simulink model "Monza"  (R2020a)
settings: Solver=FixedStepAuto  StartTime=0.0  StopTime=30  FixedStep=0.033  RelTol=1e-3
libraries: fuzblock x1, simulink x1
settings Model: Creator=jmpas  LastModifiedBy=jmpas

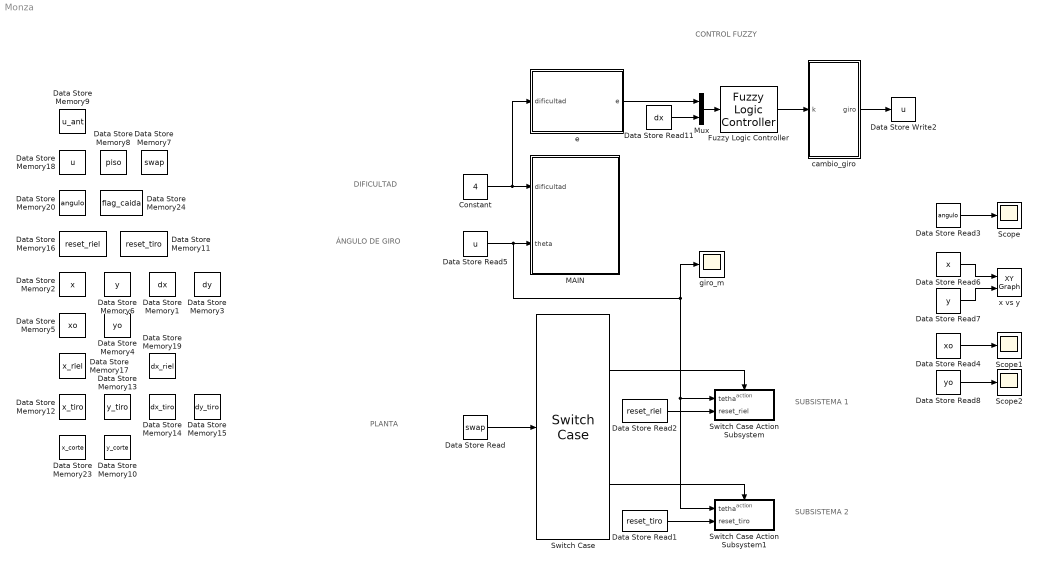
== system Monza ==
  note: CONTROL FUZZY
  note: DIFICULTAD
  note: ÁNGULO DE GIRO
  note: PLANTA
  note: SUBSISTEMA 1
  note: SUBSISTEMA 2
  " MAIN" : MATLAB Function  TreatAsAtomicUnit=on
  Constant : Constant  Value=4
  Data Store Memory1 : DataStoreMemory  DataStoreName=dx  ReadBeforeWriteMsg=warning  WriteAfterWriteMsg=warning  WriteAfterReadMsg=warning  ShowAdditionalParam=off  OutDataTypeStr=double
  Data Store Memory10 : DataStoreMemory  DataStoreName=y_corte  ReadBeforeWriteMsg=warning  WriteAfterWriteMsg=warning  WriteAfterReadMsg=warning  ShowAdditionalParam=off  OutDataTypeStr=double
  Data Store Memory11 : DataStoreMemory  DataStoreName=reset_tiro  ReadBeforeWriteMsg=warning  WriteAfterWriteMsg=warning  WriteAfterReadMsg=warning  ShowAdditionalParam=off  OutDataTypeStr=double
  Data Store Memory12 : DataStoreMemory  DataStoreName=x_tiro  ReadBeforeWriteMsg=warning  WriteAfterWriteMsg=warning  WriteAfterReadMsg=warning  ShowAdditionalParam=off  OutDataTypeStr=double
  Data Store Memory13 : DataStoreMemory  DataStoreName=y_tiro  ReadBeforeWriteMsg=warning  WriteAfterWriteMsg=warning  WriteAfterReadMsg=warning  ShowAdditionalParam=off  OutDataTypeStr=double
  Data Store Memory14 : DataStoreMemory  DataStoreName=dx_tiro  ReadBeforeWriteMsg=warning  WriteAfterWriteMsg=warning  WriteAfterReadMsg=warning  ShowAdditionalParam=off  OutDataTypeStr=double
  Data Store Memory15 : DataStoreMemory  DataStoreName=dy_tiro  ReadBeforeWriteMsg=warning  WriteAfterWriteMsg=warning  WriteAfterReadMsg=warning  ShowAdditionalParam=off  OutDataTypeStr=double
  Data Store Memory16 : DataStoreMemory  DataStoreName=reset_riel  ReadBeforeWriteMsg=warning  WriteAfterWriteMsg=warning  WriteAfterReadMsg=warning  ShowAdditionalParam=off  OutDataTypeStr=double
  Data Store Memory17 : DataStoreMemory  DataStoreName=x_riel  ReadBeforeWriteMsg=warning  WriteAfterWriteMsg=warning  WriteAfterReadMsg=warning  InitialValue=-0.11  ShowAdditionalParam=off  OutDataTypeStr=double
  Data Store Memory18 : DataStoreMemory  DataStoreName=u  ReadBeforeWriteMsg=warning  WriteAfterWriteMsg=warning  WriteAfterReadMsg=warning  InitialValue=-0.25  ShowAdditionalParam=off  OutDataTypeStr=double
  Data Store Memory19 : DataStoreMemory  DataStoreName=dx_riel  ReadBeforeWriteMsg=warning  WriteAfterWriteMsg=warning  WriteAfterReadMsg=warning  ShowAdditionalParam=off  OutDataTypeStr=double
  Data Store Memory2 : DataStoreMemory  DataStoreName=x  ReadBeforeWriteMsg=warning  WriteAfterWriteMsg=warning  WriteAfterReadMsg=warning  InitialValue=-0.11  ShowAdditionalParam=off  OutDataTypeStr=double
  Data Store Memory20 : DataStoreMemory  DataStoreName=angulo  ReadBeforeWriteMsg=warning  WriteAfterWriteMsg=warning  WriteAfterReadMsg=warning  InitialValue=-0.25  ShowAdditionalParam=off  OutDataTypeStr=double
  Data Store Memory23 : DataStoreMemory  DataStoreName=x_corte  ReadBeforeWriteMsg=warning  WriteAfterWriteMsg=warning  WriteAfterReadMsg=warning  ShowAdditionalParam=off  OutDataTypeStr=double
  Data Store Memory24 : DataStoreMemory  DataStoreName=flag_caida  ReadBeforeWriteMsg=warning  WriteAfterWriteMsg=warning  WriteAfterReadMsg=warning  ShowAdditionalParam=off  OutDataTypeStr=double
  Data Store Memory3 : DataStoreMemory  DataStoreName=dy  ReadBeforeWriteMsg=warning  WriteAfterWriteMsg=warning  WriteAfterReadMsg=warning  ShowAdditionalParam=off  OutDataTypeStr=double
  Data Store Memory4 : DataStoreMemory  DataStoreName=yo  ReadBeforeWriteMsg=warning  WriteAfterWriteMsg=warning  WriteAfterReadMsg=warning  InitialValue=0.1092  ShowAdditionalParam=off  OutDataTypeStr=double
  Data Store Memory5 : DataStoreMemory  DataStoreName=xo  ReadBeforeWriteMsg=warning  WriteAfterWriteMsg=warning  WriteAfterReadMsg=warning  InitialValue=-0.1  ShowAdditionalParam=off  OutDataTypeStr=double
  Data Store Memory6 : DataStoreMemory  DataStoreName=y  ReadBeforeWriteMsg=warning  WriteAfterWriteMsg=warning  WriteAfterReadMsg=warning  InitialValue=0.106  ShowAdditionalParam=off  OutDataTypeStr=double
  Data Store Memory7 : DataStoreMemory  DataStoreName=swap  ReadBeforeWriteMsg=warning  WriteAfterWriteMsg=warning  WriteAfterReadMsg=warning  InitialValue=1  ShowAdditionalParam=off  OutDataTypeStr=double
  Data Store Memory8 : DataStoreMemory  DataStoreName=piso  ReadBeforeWriteMsg=warning  WriteAfterWriteMsg=warning  WriteAfterReadMsg=warning  InitialValue=1  ShowAdditionalParam=off  OutDataTypeStr=double
  Data Store Memory9 : DataStoreMemory  DataStoreName=u_ant  ReadBeforeWriteMsg=warning  WriteAfterWriteMsg=warning  WriteAfterReadMsg=warning  InitialValue=-0.25  ShowAdditionalParam=off  OutDataTypeStr=double
  Data Store Read : DataStoreRead  DataStoreName=swap
  Data Store Read1 : DataStoreRead  DataStoreName=reset_tiro
  Data Store Read11 : DataStoreRead  DataStoreName=dx
  Data Store Read2 : DataStoreRead  DataStoreName=reset_riel
  Data Store Read3 : DataStoreRead  DataStoreName=angulo
  Data Store Read4 : DataStoreRead  DataStoreName=xo
  Data Store Read5 : DataStoreRead  DataStoreName=u
  Data Store Read6 : DataStoreRead  DataStoreName=x
  Data Store Read7 : DataStoreRead  DataStoreName=y
  Data Store Read8 : DataStoreRead  DataStoreName=yo
  Data Store Write2 : DataStoreWrite  DataStoreName=u
  Fuzzy Logic Controller : fuzblock/Fuzzy Logic  Controller  FIS='fuzzy5.fis'  OutputSampleNumber=101  DataType=double  FuzzifiedInputs=off  RuleFiringStrengths=off  RuleOutputs=off  AggregatedOutputs=off  SimulateUsing=Interpreted execution  OutOfRangeInputValueMessage=warning  NoRuleFiredMessage=warning  EmptyOutputFuzzySetMessage=warning
  Mux : Mux  Inputs=2
  Scope : Scope
  Scope1 : Scope
  Scope2 : Scope
  Switch Case : SwitchCase  CaseConditions={1,2}  ShowDefaultCase=off
  Switch Case Action Subsystem : Subsystem  TreatAsAtomicUnit=on
  Switch Case Action Subsystem1 : Subsystem  TreatAsAtomicUnit=on
  cambio_giro : MATLAB Function  TreatAsAtomicUnit=on
  e : MATLAB Function  TreatAsAtomicUnit=on
  giro_m : Scope
  x vs y : simulink/Sinks/XY Graph  xmin=-0.5  xmax=0.5  ymin=-0.2  ymax=0.2  st=-1
  wires:
  Switch Case/1 -> Switch Case Action Subsystem/Action
  cambio_giro/1(giro) -> Data Store Write2/1
  Data Store Read5/1 -> " MAIN"/2(theta), Switch Case Action Subsystem/1(tetha), Switch Case Action Subsystem1/1(tetha), giro_m/1
  Switch Case/2 -> Switch Case Action Subsystem1/Action
  Fuzzy Logic Controller/1 -> cambio_giro/1(k)
  Data Store Read/1 -> Switch Case/1
  Data Store Read1/1 -> Switch Case Action Subsystem1/2(reset_tiro)
  Data Store Read2/1 -> Switch Case Action Subsystem/2(reset_riel)
  Mux/1 -> Fuzzy Logic Controller/1
  Constant/1 -> e/1(dificultad), " MAIN"/1(dificultad)
  e/1(e) -> Mux/1
  Data Store Read11/1 -> Mux/2
  Data Store Read7/1 -> x vs y/2
  Data Store Read4/1 -> Scope1/1
  Data Store Read6/1 -> x vs y/1
  Data Store Read3/1 -> Scope/1
  Data Store Read8/1 -> Scope2/1

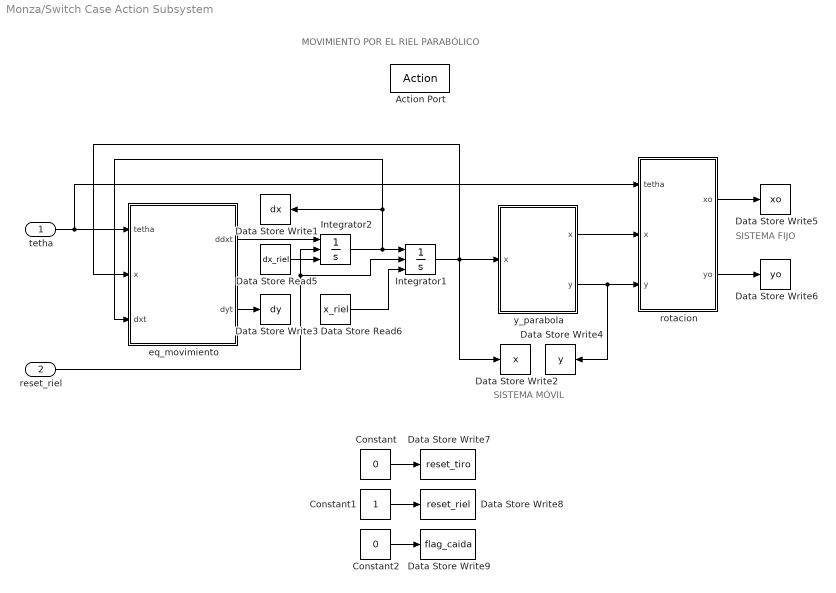
== system Monza/Switch Case Action Subsystem ==
  note: SISTEMA FIJO
  note: SISTEMA MÓVIL
  note: MOVIMIENTO POR EL RIEL PARABÓLICO
  tetha : Inport
  reset_riel : Inport  Port=2
  Action Port : ActionPort  ActionPortLabel=case [ 1 ]:
  " y_parabola" : MATLAB Function  TreatAsAtomicUnit=on
  Constant : Constant  Value=0
  Constant1 : Constant
  Constant2 : Constant  Value=0
  Data Store Read5 : DataStoreRead  DataStoreName=dx_riel
  Data Store Read6 : DataStoreRead  DataStoreName=x_riel
  Data Store Write1 : DataStoreWrite  DataStoreName=dx
  Data Store Write2 : DataStoreWrite  DataStoreName=x
  Data Store Write3 : DataStoreWrite  DataStoreName=dy
  Data Store Write4 : DataStoreWrite  DataStoreName=y
  Data Store Write5 : DataStoreWrite  DataStoreName=xo
  Data Store Write6 : DataStoreWrite  DataStoreName=yo
  Data Store Write7 : DataStoreWrite  DataStoreName=reset_tiro
  Data Store Write8 : DataStoreWrite  DataStoreName=reset_riel
  Data Store Write9 : DataStoreWrite  DataStoreName=flag_caida
  Integrator1 : Integrator  ExternalReset=falling  InitialConditionSource=external
  Integrator2 : Integrator  ExternalReset=falling  InitialConditionSource=external
  eq_movimiento : MATLAB Function  TreatAsAtomicUnit=on
  rotacion : MATLAB Function  TreatAsAtomicUnit=on
  wires:
  tetha/1 -> eq_movimiento/1(tetha), rotacion/1(tetha)
  " y_parabola"/2(y) -> rotacion/3(y), Data Store Write4/1
  Integrator1/1 -> eq_movimiento/2(x), Data Store Write2/1, " y_parabola"/1("x ")
  " y_parabola"/1(x) -> rotacion/2(x)
  Integrator2/1 -> Integrator1/1, eq_movimiento/3(dxt), Data Store Write1/1
  rotacion/2(yo) -> Data Store Write6/1
  rotacion/1(xo) -> Data Store Write5/1
  reset_riel/1 -> Integrator1/2, Integrator2/2
  Data Store Read5/1 -> Integrator2/3
  Data Store Read6/1 -> Integrator1/3
  eq_movimiento/2(dyt) -> Data Store Write3/1
  eq_movimiento/1(ddxt) -> Integrator2/1
  Constant/1 -> Data Store Write7/1
  Constant1/1 -> Data Store Write8/1
  Constant2/1 -> Data Store Write9/1

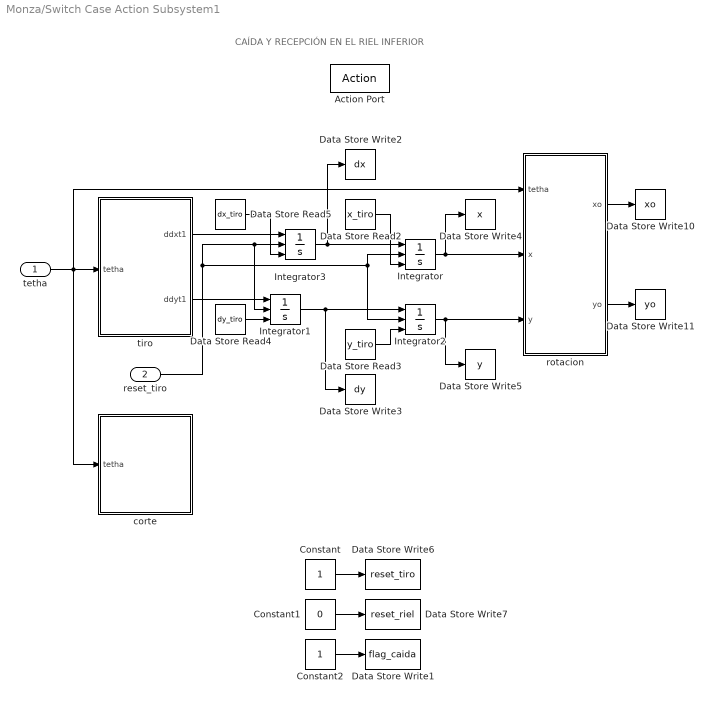
== system Monza/Switch Case Action Subsystem1 ==
  note: CAÍDA Y RECEPCIÓN EN EL RIEL INFERIOR
  tetha : Inport
  reset_tiro : Inport  Port=2
  Action Port : ActionPort  ActionPortLabel=case [ 2 ]:
  Constant : Constant
  Constant1 : Constant  Value=0
  Constant2 : Constant
  Data Store Read2 : DataStoreRead  DataStoreName=x_tiro
  Data Store Read3 : DataStoreRead  DataStoreName=y_tiro
  Data Store Read4 : DataStoreRead  DataStoreName=dy_tiro
  Data Store Read5 : DataStoreRead  DataStoreName=dx_tiro
  Data Store Write1 : DataStoreWrite  DataStoreName=flag_caida
  Data Store Write10 : DataStoreWrite  DataStoreName=xo
  Data Store Write11 : DataStoreWrite  DataStoreName=yo
  Data Store Write2 : DataStoreWrite  DataStoreName=dx
  Data Store Write3 : DataStoreWrite  DataStoreName=dy
  Data Store Write4 : DataStoreWrite  DataStoreName=x
  Data Store Write5 : DataStoreWrite  DataStoreName=y
  Data Store Write6 : DataStoreWrite  DataStoreName=reset_tiro
  Data Store Write7 : DataStoreWrite  DataStoreName=reset_riel
  Integrator{,1..3} (4 alike) : Integrator  ExternalReset=falling  InitialConditionSource=external
  corte : MATLAB Function  TreatAsAtomicUnit=on
  rotacion : MATLAB Function  TreatAsAtomicUnit=on
  tiro : MATLAB Function  TreatAsAtomicUnit=on
  wires:
  tiro/1(ddxt1) -> Integrator3/1
  tiro/2(ddyt1) -> Integrator1/1
  Integrator3/1 -> Integrator/1, Data Store Write2/1
  Integrator1/1 -> Integrator2/1, Data Store Write3/1
  Integrator/1 -> Data Store Write4/1, rotacion/2(x)
  Integrator2/1 -> Data Store Write5/1, rotacion/3(y)
  reset_tiro/1 -> Integrator2/2, Integrator/2, Integrator3/2, Integrator1/2
  Data Store Read4/1 -> Integrator1/3
  Data Store Read5/1 -> Integrator3/3
  Data Store Read2/1 -> Integrator/3
  Data Store Read3/1 -> Integrator2/3
  Constant/1 -> Data Store Write6/1
  Constant1/1 -> Data Store Write7/1
  tetha/1 -> corte/1(tetha), tiro/1(tetha), rotacion/1(tetha)
  rotacion/1(xo) -> Data Store Write10/1
  rotacion/2(yo) -> Data Store Write11/1
  Constant2/1 -> Data Store Write1/1

== matlab function Monza/Switch Case Action Subsystem1/tiro ==
  settings: updateMethod=DISCRETE
  data: ddxt1 output; ddyt1 output; tetha input
function [ddxt1, ddyt1] = fcn(tetha)
g = 9.81;
ddxt1 = -g*sin(tetha);
ddyt1 = -g*cos(tetha);
end

== matlab function Monza/Switch Case Action Subsystem/rotacion ==
  data: xo output; yo output; tetha input; x input; y input
function [xo,yo] = fcn(tetha,x,y)
xo=x*cos(tetha)-y*sin(tetha);
yo=x*sin(tetha)+y*cos(tetha);
end

== matlab function Monza/Switch Case Action Subsystem1/corte ==
  settings: updateMethod=DISCRETE
  data: piso data_store_memory; x data_store_memory; y data_store_memory; tetha input; dx data_store_memory; dy data_store_memory; x_corte data_store_memory; y_corte data_store_memory; x_tiro data_store_memory; y_tiro data_store_memory; dx_tiro data_store_memory; dy_tiro data_store_memory; flag_caida data_store_memory
function fcn(tetha)

coder.extrinsic('corte');

global piso

global x_corte
global y_corte
global x_tiro
global y_tiro
global dx_tiro
global dy_tiro
global flag_caida

[x_corte,y_corte] = corte(tetha,piso,x_tiro,y_tiro,dx_tiro,dy_tiro,flag_caida);

end

== matlab function Monza/Switch Case Action Subsystem1/rotacion ==
  data: xo output; yo output; tetha input; x input; y input
function [xo,yo] = fcn(tetha,x,y)
xo=x*cos(tetha)-y*sin(tetha);
yo=x*sin(tetha)+y*cos(tetha);
end

== matlab function Monza/cambio_giro ==
  settings: updateMethod=DISCRETE
  data: k input; giro output; angulo data_store_memory; piso data_store_memory; u_ant data_store_memory
function giro = fcn(k)
global u_ant

%Nuevo giro
%El anterior más la ganancia del controlador
giro = u_ant + k;

%Saturación giro 60º
if (giro < -1)
    
    giro = -1;

elseif(giro > 1)
    
    giro = 1;
    
end
end

== matlab function Monza/e ==
  settings: updateMethod=DISCRETE
  data: e output; piso data_store_memory; x data_store_memory; dificultad input
function e = fcn(dificultad)
coder.extrinsic('finalRiel');
global piso
global x 

%Inicializa finales de riel:
x1d = 0;
x2i = 0;
x3d = 0;
x4i = 0;
x5d = 0; 
x6i = 0;
x7d = 0;

%Se cargan los finales según la dificultad
[x1d,x2i,x3d,x4i,x5d,x6i,x7d] = finalRiel(dificultad);

%Inicializo el error
%Diferencia entre donde quiero llegar y donde estoy
e = 0.11;

switch piso

    case 1
        e = x1d-x;
    case 2
        e = x2i-x;
    case 3
        e = x3d-x;
    case 4
        e = x4i-x;
    case 5
        e = x5d-x;
    case 6
        e = x6i-x;
    case 7
        e = x7d-x;
        
end

== matlab function Monza/Switch Case Action Subsystem/ y_parabola ==
  settings: updateMethod=DISCRETE
  data: x output; x input; y output; piso data_store_memory
function [x,y] = fcn(x)
global piso
y=0;
switch piso
    case 1
        y = -0.54*x^2+0.1143;
    case 2
        y = -0.54*x^2+0.0686;
    case 3
        y = -0.54*x^2+0.0229;
    case 4
        y = -0.54*x^2-0.0229;
    case 5
        y = -0.54*x^2-0.0686;
    case 6
        y = -0.54*x^2-0.1143; 
    case 7
        y = -0.54*x^2-0.16;
end

== matlab function Monza/Switch Case Action Subsystem/eq_movimiento ==
  data: tetha input; ddxt output; x input; dxt input; dyt output
function [ddxt, dyt] = fcn(tetha,x,dxt)
g = 9.81;
m = 0.007; %50cents
c = 0.01; %coeficiente viscoso

%beta = atan(1.08*x);
%ddxt = (2/3)*g*sin(beta-theta);
ddxt = (m*g*-sin(atan(-1.08*x)+tetha)-c*dxt)/m;
dyt = -1.08*x*dxt;
end

== matlab function Monza/ MAIN ==
  settings: updateMethod=DISCRETE
  data: dificultad input; theta input; x data_store_memory; y data_store_memory; dx data_store_memory; piso data_store_memory; swap data_store_memory; reset_tiro data_store_memory; x_tiro data_store_memory; y_tiro data_store_memory; dx_tiro data_store_memory; dy_tiro data_store_memory; reset_riel data_store_memory; x_riel data_store_memory; dx_riel data_store_memory; dy data_store_memory; angulo data_store_memory; x_corte data_store_memory; y_corte data_store_memory; flag_caida data_store_memory; xo data_store_memory; yo data_store_memory; u_ant data_store_memory
function fcn(dificultad,theta)
coder.extrinsic('gcs');
coder.extrinsic('set_param');
coder.extrinsic('finalRiel');
global piso
global swap

global angulo
global u_ant

global x
global y
global xo
global yo

global dx
global dy

global x_riel
global dx_riel
global reset_riel

global x_tiro
global y_tiro
global dx_tiro
global dy_tiro
global reset_tiro

global x_corte
global y_corte
global flag_caida

aux=0;

u_ant = theta;

%Ángulo moneda
if piso == 1 || piso == 2 || piso == 3
    angulo = atan(yo/xo);
elseif piso == 4 || piso == 5 || piso == 6
    angulo = -atan(yo/xo);
end

%Inicialización
x1d = 0;
x2i = 0;
x3d = 0;
x4i = 0;
x5d = 0; 
x6i = 0;
x7d = 0;

%************************* DIFICULTAD ********************************** 

[x1d,x2i,x3d,x4i,x5d,x6i,x7d] = finalRiel(dificultad);
  
%************************* MOVIMIENTO RIEL ***************************** 
%la moneda se mueve sobre el riel parabólico
if swap == 1
    
    reset_riel = 1;
    flag_caida = 0;
    
    switch piso
        case 1
            if x >= x1d %si sobrepasa el extremo del riel
                swap = 2; %va a caer
                aux = 1;
                reset_tiro = 0;
            end
        case 2
            if x <= x2i
                swap = 2;
                aux = 1;
                reset_tiro = 0;                
            end
        case 3
            if x >= x3d
                swap = 2;
                aux = 1;
                reset_tiro = 0;
            end
        case 4
            if x <= x4i
                swap = 2;
                aux = 1;
                reset_tiro = 0;                
            end
        case 5
            if x >= x5d
                swap = 2;
                aux = 1;
                reset_tiro = 0;
            end
        case 6
            if x <= x6i
                swap = 2;
                aux = 1;
                reset_tiro = 0;                
            end
        case 7
            if x >= x7d
%                 swap = 2;
%                 aux = 1;
%                 reset_tiro = 0;   
                set_param(gcs, 'SimulationCommand', 'stop')
            end
    end
    
    if aux == 1         %la moneda va a caer
        
        dx_tiro = dx;  %preparo datos para el tiro
        dy_tiro = dy;
        x_tiro = x;
        y_tiro = y;
        
    end
    
%************************* TIRO ****************************************   

elseif swap == 2    
        
        reset_tiro = 1;
        flag_caida = 1;
        
        if y<=y_corte
            
%             v = 0;
%             alpha = 0;
            piso = piso + 1;    %cambio de piso
            reset_riel = 0;
            
            x_riel = x_corte; %dónde ha caido?
%             v = sqrt(dx^2+dy^2);
%             alpha = atan(dy/dx);
%             beta = atan(1.08*x_corte);
%             dx_riel = v*cos(beta - alpha)*cos(beta);
            dx_riel = dx;
            swap = 1;   %vuelve a moverse sobre el riel
        
        end
end
